simulink model "FOC_V"  (R2016b)
settings: Solver=VariableStepAuto  StartTime=0.0  StopTime=5  FixedStep=1e-6  RelTol=1e-3  EnableMultiTasking=on
model workspace (MAT data in the model file):
  Cf = 1e-05
  J = 0.02
  Lf = 0.005
  Lm = 0.27325
  Lr = 0.289368
  Ls = 0.289368
  P = 4
  Rf = 5
  Rr = 3.3278
  Rs = 4.6
  Sig = Simulink.Signal
  Sig.DataType = 'auto'
  Sig.Dimensions = -1
  Sig.DimensionsMode = 'auto'
  Sig.Complexity = 'auto'
  Sig.SampleTime = -1
  Sig.SamplingMode = 'auto'
  Ts = 0.0001
  idth = 1.6
  nth = 370
  theta0 = 0
libraries: powerlib x15, simulink x8
settings Model: Creator=yoush  LastModifiedBy=yoush
settings DataIOCC: LimitDataPoints=on
settings OptimizationCC: LifeSpan=inf
settings DebuggingCC: AllowSymbolicDim=off  SFUnexpectedBacktrackingDiag=warning  SFNoUnconditionalDefaultTransitionDiag=warning  SFExecutionAtInitializationDiag=none
settings ModelReferenceCC: PropagateSignalLabelsOutOfModel=off
settings GRTTargetCC: TargetLangStandard=C89/C90 (ANSI)
settings ConfigComp: CovMetricSettings=dw  CovHtmlReporting=on  CovSaveCumulativeToWorkspaceVar=on  CovSaveSingleToWorkspaceVar=on  CovExternalEMLEnable=off
settings ConfigurationSet: Description=SimMechanics 2G

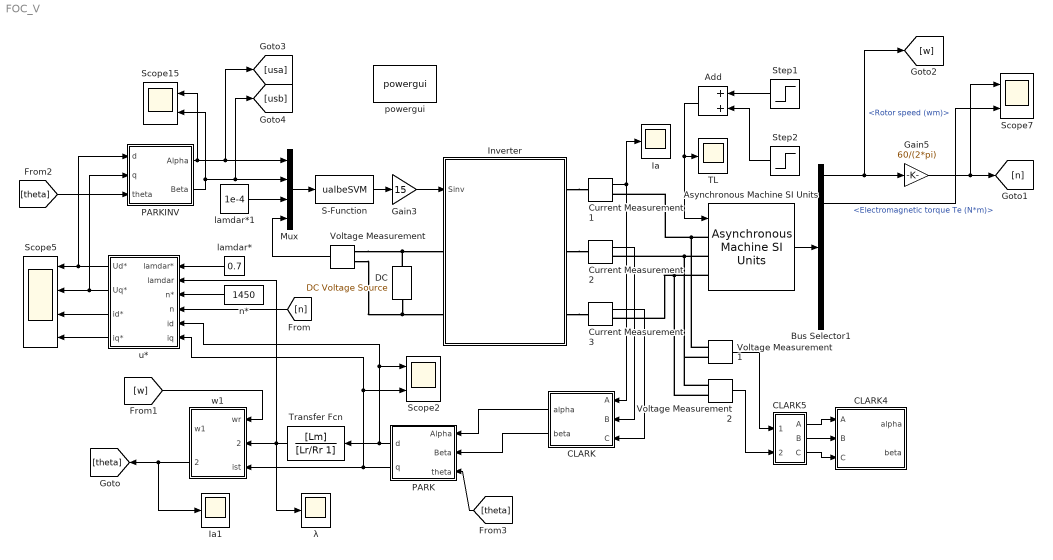
== system FOC_V ==
  Add : Sum
  Asynchronous Machine SI Units : powerlib/Machines/Asynchronous Machine SI Units  RotorType=Squirrel-cage  PresetModel=No  MechanicalLoad=Torque Tm  ShowDetailedParameters=on  ReferenceFrame=Rotor  Units=SI  MeasurementBus=off  NominalParameters=[22000 380 50]  Stator=[4.6 0.016118]  Rotor=[3.3278 0.016118]  Cage1=[0.4155 0.002066]  Cage2=[0.4168 0.0003495]  Lm=0.27325  Mechanical=[0.02 0 2]  PolePairs=2  InitialConditions=[ 1 0 0 0 0 0 0 0]  SimulateSaturation=off  Saturation=[14.03593122, 27.81365428, 53.79336849, 72.68890987, 97.98006896, 148.6815601, 215.7428561, 302.9841135, 428.7778367 ; 230, 322, 414, 460, 506, 552, 598, 644, 690]  LoadFlowParameters=1492000  TsPowergui=0  TsBlock=-1  IterativeModel=Trapezoidal non iterative  IterativeDiscreteModel=Trapezoidal non iterative  Pmec=1.492e+006
  Bus Selector1 : BusSelector  OutputSignals="Mechanical.Rotor speed (wm),Mechanical.Electromagnetic torque Te (N*m),Stator measurements.Stator current is_d (A),Stator measurements.Stator current  is_q (A),Rotor measurements.Rotor flux phir_q (V s),Rotor measurements.Rotor flux phir_d (V s)"
  CLARK : Subsystem
  CLARK4 : Subsystem
  CLARK5 : Subsystem
  Current Measurement1 : powerlib/Measurements/Current Measurement  PhasorSimulation=off  OutputType=Complex  PSBequivalent=0
  Current Measurement2 : powerlib/Measurements/Current Measurement  PhasorSimulation=off  OutputType=Complex  PSBequivalent=0
  Current Measurement3 : powerlib/Measurements/Current Measurement  PhasorSimulation=off  OutputType=Complex  PSBequivalent=0
  DC : powerlib/Electrical Sources/DC Voltage Source  Amplitude=500  Measurements=None
  Gain3 : Gain  Gain=15
  Gain5 : Gain  Gain=60/(2*pi)
  Ia : Scope
  Ia1 : Scope
  Inverter : Subsystem
  Mux : Mux
  PARK : Subsystem
  PARKINV : Subsystem
  S-Function : S-Function  FunctionName=ualbeSVM  SFunctionDeploymentMode=off  EnableBusSupport=off
  Scope15 : Scope  NumInputPorts=2
  Scope2 : Scope  NumInputPorts=2
  Scope5 : Scope  NumInputPorts=4
  Scope7 : Scope  NumInputPorts=2
  Step1 : Step  Time=2  After=2  SampleTime=0
  Step2 : Step  Time=5  After=0  SampleTime=0
  TL : Scope
  Transfer Fcn : TransferFcn  Numerator=[Lm]  Denominator=[Lr/Rr 1]
  Voltage Measurement : powerlib/Measurements/Voltage Measurement  PhasorSimulation=off  OutputType=Complex  PSBequivalent=0
  Voltage Measurement1 : powerlib/Measurements/Voltage Measurement  PhasorSimulation=off  OutputType=Complex  PSBequivalent=0
  Voltage Measurement2 : powerlib/Measurements/Voltage Measurement  PhasorSimulation=off  OutputType=Complex  PSBequivalent=0
  lamdar* : Constant  Value=0.7
  lamdar*1 : Constant  Value=1e-4
  n* : Constant  Value=1450
  powergui : powerlib/powergui  Priority=1  SimulationMode=Continuous  SolverType=Tustin/Backward Euler (TBE)  SampleTime=1e-6  frequency=60  SPID=off  DisableSnubberDevices=off  DisableRonSwitches=off  DisableVfSwitches=off  SwTol=0  DisplayEquations=off  Interpol=off  ExternalGateDelay=off  methode=off  Ts=10  FunctionMessages=off  echomessages=off  HookPort=off  EnableUseOfTLC=off  x0status=blocks  frequencyindice=50  Pbase=100e6  ErrMax=1e-4  Iterations=50  UnitsV=kV  UnitsW=MW  buscounter=0  RestoreLinks=warning  ResistiveCurrentMeasurement=off  Frange=[0:2:500]  Ylog=off  Xlog=on  ShowGrid=off  save=off  variable=ZData  structure=we  ZoomFFT=off  StartTime=0.4  cycles=5  DisplayStyle=2  fundamental=100  FreqAxis=off  MaxFrequency=1000  frequencyindicesteady=1  RmsSteady=1  display=off
  u* : Subsystem
  w1 : Subsystem
  λ : Scope
  wires:
  Current Measurement1/1 -> CLARK/1(A), Ia/1
  Add/1 -> Asynchronous Machine SI Units/1, TL/1
  Step1/1 -> Add/1
  Step2/1 -> Add/2
  Asynchronous Machine SI Units/1 -> Bus Selector1/1
  Bus Selector1/1 -> Gain5/1, [w]  "<Rotor speed (wm)>"
  Gain5/1 -> [n], Scope7/1
  Bus Selector1/2 -> Scope7/2  "<Electromagnetic torque Te (N*m)>"
  Current Measurement2/1 -> CLARK/2(B)
  Current Measurement3/1 -> CLARK/3(C)
  CLARK/1(alpha) -> PARK/1(Alpha)
  CLARK/2(beta) -> PARK/2(Beta)
  PARK/2(q) -> Scope2/2, u*/6(iq), w1/3(ist)
  [n] -> u*/4(n)
  Gain3/1 -> Inverter/1(Sinv)
  lamdar*/1 -> u*/1(lamdar*)
  n*/1 -> u*/3(n*)
  PARK/1(d) -> Transfer Fcn/1, Scope2/1, u*/5(id)
  PARKINV/1(Alpha) -> [usa], Mux/1, Scope15/1
  PARKINV/2(Beta) -> [usb], Mux/2, Scope15/2
  [theta] -> PARKINV/3(theta)
  [theta] -> PARK/3(theta)
  u*/1(Ud*) -> Scope5/1, PARKINV/1(d)
  u*/2(Uq*) -> PARKINV/2(q), Scope5/2
  Mux/1 -> S-Function/1
  lamdar*1/1 -> Mux/3
  Voltage Measurement/1 -> Mux/4
  S-Function/1 -> Gain3/1
  Transfer Fcn/1 -> λ/1, w1/2(lamdar), u*/2(lamdar)
  [w] -> w1/1(wr)
  u*/3(id*) -> Scope5/3
  w1/2(theta) -> [theta], Ia1/1
  u*/4(iq*) -> Scope5/4
  Voltage Measurement1/1 -> CLARK5/1(AB)
  Voltage Measurement2/1 -> CLARK5/2(BC)
  CLARK5/2(B) -> CLARK4/2(B)
  CLARK5/1(A) -> CLARK4/1(A)
  CLARK5/3(C) -> CLARK4/3(C)
  connections:
  Inverter/RConn1 -- Current Measurement1/LConn1
  Inverter/RConn2 -- Current Measurement2/LConn1
  Inverter/RConn3 -- Current Measurement3/LConn1
  Asynchronous Machine SI Units/LConn1 -- Voltage Measurement1/LConn1 -- Current Measurement1/RConn1
  Asynchronous Machine SI Units/LConn2 -- Voltage Measurement2/LConn1 -- Voltage Measurement1/LConn2 -- Current Measurement2/RConn1
  Asynchronous Machine SI Units/LConn3 -- Voltage Measurement2/LConn2 -- Current Measurement3/RConn1
  DC/RConn1 -- Voltage Measurement/LConn1 -- Inverter/LConn1
  DC/LConn1 -- Voltage Measurement/LConn2 -- Inverter/LConn2

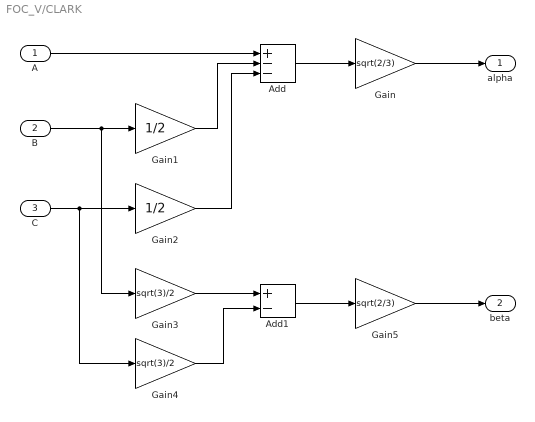
== system FOC_V/CLARK ==
  A : Inport
  B : Inport  Port=2
  C : Inport  Port=3
  Add : Sum  Inputs=+--
  Add1 : Sum  Inputs=+-
  Gain : Gain  Gain=sqrt(2/3)
  Gain1 : Gain  Gain=1/2
  Gain2 : Gain  Gain=1/2
  Gain3 : Gain  Gain=sqrt(3)/2
  Gain4 : Gain  Gain=sqrt(3)/2
  Gain5 : Gain  Gain=sqrt(2/3)
  alpha : Outport
  beta : Outport  Port=2
  wires:
  A/1 -> Add/1
  B/1 -> Gain3/1, Gain1/1
  Gain1/1 -> Add/2
  Gain2/1 -> Add/3
  C/1 -> Gain4/1, Gain2/1
  Gain3/1 -> Add1/1
  Gain4/1 -> Add1/2
  Add/1 -> Gain/1
  Add1/1 -> Gain5/1
  Gain/1 -> alpha/1
  Gain5/1 -> beta/1

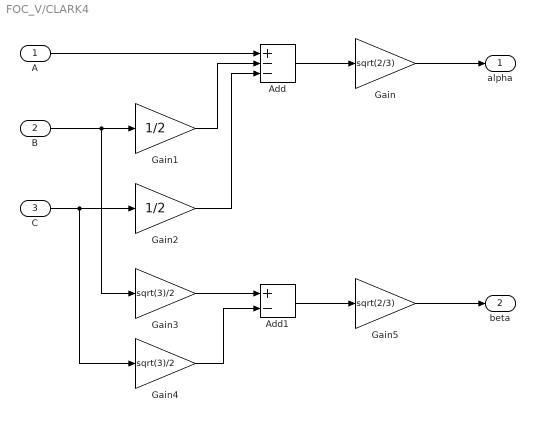
== system FOC_V/CLARK4 ==
  A : Inport
  B : Inport  Port=2
  C : Inport  Port=3
  Add : Sum  Inputs=+--
  Add1 : Sum  Inputs=+-
  Gain : Gain  Gain=sqrt(2/3)
  Gain1 : Gain  Gain=1/2
  Gain2 : Gain  Gain=1/2
  Gain3 : Gain  Gain=sqrt(3)/2
  Gain4 : Gain  Gain=sqrt(3)/2
  Gain5 : Gain  Gain=sqrt(2/3)
  alpha : Outport
  beta : Outport  Port=2
  wires:
  Gain5/1 -> beta/1
  Gain/1 -> alpha/1
  Add1/1 -> Gain5/1
  Add/1 -> Gain/1
  Gain4/1 -> Add1/2
  Gain3/1 -> Add1/1
  C/1 -> Gain2/1, Gain4/1
  Gain2/1 -> Add/3
  Gain1/1 -> Add/2
  B/1 -> Gain1/1, Gain3/1
  A/1 -> Add/1

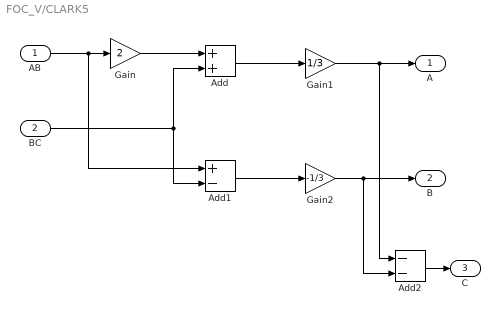
== system FOC_V/CLARK5 ==
  AB : Inport
  BC : Inport  Port=2
  Add : Sum
  Add1 : Sum  Inputs=+-
  Add2 : Sum  Inputs=--
  Gain : Gain  Gain=2
  Gain1 : Gain  Gain=1/3
  Gain2 : Gain  Gain=-1/3
  A : Outport
  B : Outport  Port=2
  C : Outport  Port=3
  wires:
  AB/1 -> Add1/1, Gain/1
  Gain/1 -> Add/1
  BC/1 -> Add/2, Add1/2
  Add/1 -> Gain1/1
  Gain1/1 -> Add2/1, A/1
  Add1/1 -> Gain2/1
  Gain2/1 -> Add2/2, B/1
  Add2/1 -> C/1

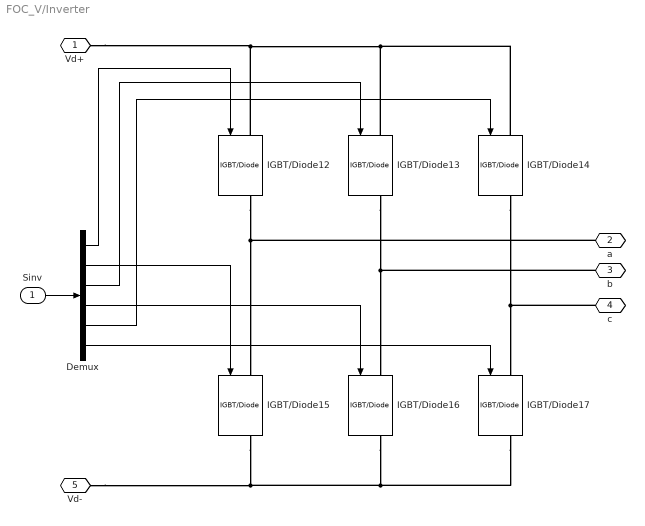
== system FOC_V/Inverter ==
  Sinv : Inport
  Demux : Demux  Outputs=6
  IGBT/Diode{12..17} (6 alike) : powerlib/Power Electronics/IGBT//Diode  Ron=1e-3  Rs=1e5  Cs=inf  Measurements=on
  Vd+ : PMIOPort  Port=1  Side=Left
  a : PMIOPort  Port=2  Side=Right
  b : PMIOPort  Port=3  Side=Right
  c : PMIOPort  Port=4  Side=Right
  Vd- : PMIOPort  Port=5  Side=Left
  wires:
  Demux/5 -> IGBT/Diode14/1
  Demux/4 -> IGBT/Diode16/1
  Demux/3 -> IGBT/Diode13/1
  Demux/6 -> IGBT/Diode17/1
  Demux/1 -> IGBT/Diode12/1
  Sinv/1 -> Demux/1
  Demux/2 -> IGBT/Diode15/1
  connections:
  IGBT/Diode12/RConn1 -- IGBT/Diode15/LConn1 -- a/RConn1
  IGBT/Diode13/RConn1 -- IGBT/Diode16/LConn1 -- b/RConn1
  IGBT/Diode14/RConn1 -- IGBT/Diode17/LConn1 -- c/RConn1
  IGBT/Diode17/RConn1 -- IGBT/Diode16/RConn1 -- Vd-/RConn1 -- IGBT/Diode15/RConn1
  IGBT/Diode12/LConn1 -- Vd+/RConn1 -- IGBT/Diode13/LConn1 -- IGBT/Diode14/LConn1

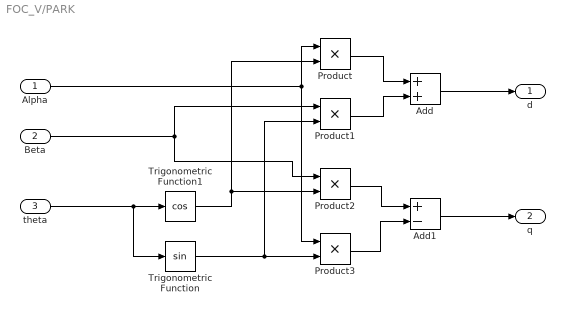
== system FOC_V/PARK ==
  Alpha : Inport
  Beta : Inport  Port=2
  theta : Inport  Port=3
  Add : Sum
  Add1 : Sum  Inputs=+-
  Product{,1..3} (4 alike) : Product
  Trigonometric Function : Trigonometry
  Trigonometric Function1 : Trigonometry  Operator=cos
  d : Outport
  q : Outport  Port=2
  wires:
  theta/1 -> Trigonometric Function1/1, Trigonometric Function/1
  Trigonometric Function1/1 -> Product/2, Product2/2
  Alpha/1 -> Product/1, Product3/1
  Trigonometric Function/1 -> Product1/2, Product3/2
  Beta/1 -> Product2/1, Product1/1
  Product/1 -> Add/1
  Product1/1 -> Add/2
  Add/1 -> d/1
  Product2/1 -> Add1/1
  Product3/1 -> Add1/2
  Add1/1 -> q/1

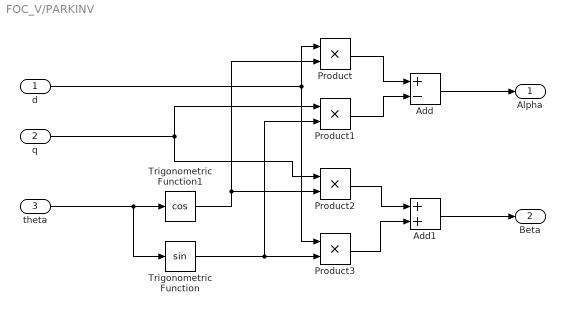
== system FOC_V/PARKINV ==
  d : Inport
  q : Inport  Port=2
  theta : Inport  Port=3
  Add : Sum  Inputs=+-
  Add1 : Sum
  Product{,1..3} (4 alike) : Product
  Trigonometric Function : Trigonometry
  Trigonometric Function1 : Trigonometry  Operator=cos
  Alpha : Outport
  Beta : Outport  Port=2
  wires:
  theta/1 -> Trigonometric Function1/1, Trigonometric Function/1
  Trigonometric Function1/1 -> Product/2, Product2/2
  d/1 -> Product/1, Product3/1
  Trigonometric Function/1 -> Product1/2, Product3/2
  q/1 -> Product2/1, Product1/1
  Product/1 -> Add/1
  Product1/1 -> Add/2
  Add/1 -> Alpha/1
  Product2/1 -> Add1/1
  Product3/1 -> Add1/2
  Add1/1 -> Beta/1

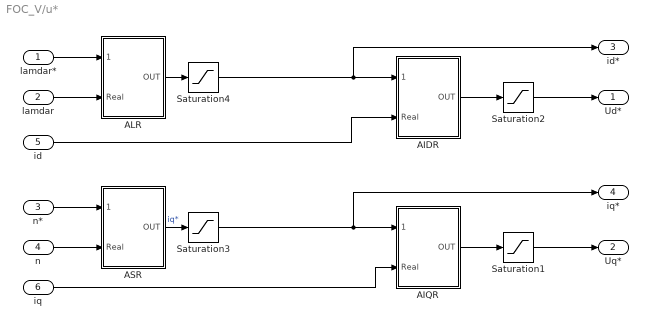
== system FOC_V/u* ==
  lamdar* : Inport
  lamdar : Inport  Port=2
  n* : Inport  Port=3
  n : Inport  Port=4
  id : Inport  Port=5
  iq : Inport  Port=6
  AIDR : Subsystem
  AIQR : Subsystem
  ALR : Subsystem
  ASR : Subsystem
  Saturation1 : Saturate  UpperLimit=380  LowerLimit=-380
  Saturation2 : Saturate  UpperLimit=380  LowerLimit=-380
  Saturation3 : Saturate  UpperLimit=5  LowerLimit=-5
  Saturation4 : Saturate  UpperLimit=5  LowerLimit=-5
  Ud* : Outport
  Uq* : Outport  Port=2
  id* : Outport  Port=3
  iq* : Outport  Port=4
  wires:
  lamdar*/1 -> ALR/1(Command)
  lamdar/1 -> ALR/2(Real)
  n*/1 -> ASR/1(Command)
  n/1 -> ASR/2(Real)
  Saturation1/1 -> Uq*/1
  Saturation2/1 -> Ud*/1
  ASR/1(OUT) -> Saturation3/1  "iq*"
  AIQR/1(OUT) -> Saturation1/1
  iq/1 -> AIQR/2(Real)
  ALR/1(OUT) -> Saturation4/1
  id/1 -> AIDR/2(Real)
  AIDR/1(OUT) -> Saturation2/1
  Saturation3/1 -> iq*/1, AIQR/1(Command)
  Saturation4/1 -> id*/1, AIDR/1(Command)

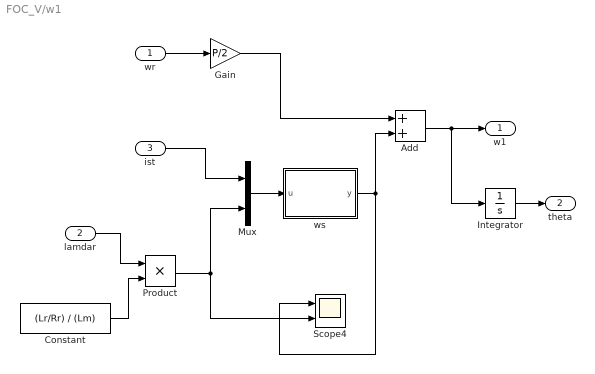
== system FOC_V/w1 ==
  wr : Inport
  lamdar : Inport  Port=2
  ist : Inport  Port=3
  Add : Sum
  Constant : Constant  Value=(Lr/Rr) / (Lm)
  Gain : Gain  Gain=P/2
  Integrator : Integrator
  Mux : Mux  Inputs=2
  Product : Product
  Scope4 : Scope  NumInputPorts=2
  ws : MATLAB Function  TreatAsAtomicUnit=on
  w1 : Outport
  theta : Outport  Port=2
  wires:
  ist/1 -> Mux/1
  Mux/1 -> ws/1(u)
  ws/1(y) -> Scope4/1, Add/2
  wr/1 -> Gain/1
  Add/1 -> Integrator/1, w1/1
  Gain/1 -> Add/1
  lamdar/1 -> Product/1
  Constant/1 -> Product/2
  Product/1 -> Mux/2, Scope4/2
  Integrator/1 -> theta/1

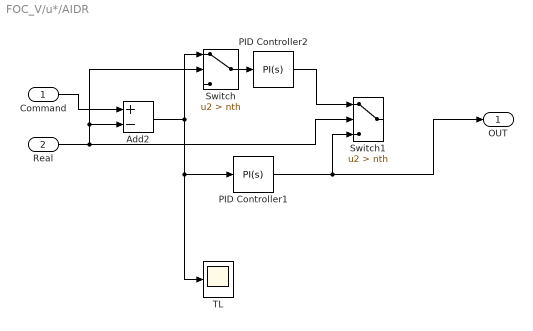
== system FOC_V/u*/AIDR ==
  Command : Inport
  Real : Inport  Port=2
  Add2 : Sum  Inputs=+-
  PID Controller1 : simulink/Continuous/PID Controller  Controller=PI  TimeDomain=Continuous-time  SampleTime=-1  IntegratorMethod=Forward Euler  FilterMethod=Forward Euler  Form=Parallel  UseFilter=on  ControllerParametersSource=internal  P=100  I=1500  D=0  N=100  InitialConditionSource=internal  InitialConditionForIntegrator=0  InitialConditionForFilter=0  ExternalReset=none  LimitOutput=off  UpperSaturationLimit=inf  LowerSaturationLimit=-inf  LinearizeAsGain=on  AntiWindupMode=none  Kb=1  TrackingMode=off  Kt=1  PParamMin=[]  PParamMax=[]  IParamMin=[]  IParamMax=[]  DParamMin=[]  DParamMax=[]  NParamMin=[]  NParamMax=[]  KbParamMin=[]  KbParamMax=[]  KtParamMin=[]  KtParamMax=[]  POutMin=[]  POutMax=[]  IOutMin=[]  IOutMax=[]  DOutMin=[]  DOutMax=[]  NOutMin=[]  NOutMax=[]  KbOutMin=[]  KbOutMax=[]  KtOutMin=[]  KtOutMax=[]  IntegratorOutMin=[]  IntegratorOutMax=[]  FilterOutMin=[]  FilterOutMax=[]  SumOutMin=[]  SumOutMax=[]  SumI1OutMin=[]  SumI1OutMax=[]  SumI2OutMin=[]  SumI2OutMax=[]  SumI3OutMin=[]  SumI3OutMax=[]  SumDOutMin=[]  SumDOutMax=[]  SaturationOutMin=[]  SaturationOutMax=[]  IntegratorContinuousStateAttributes=''  IntegratorStateMustResolveToSignalObject=off  IntegratorRTWStateStorageClass=Auto  FilterContinuousStateAttributes=''  FilterStateMustResolveToSignalObject=off  FilterRTWStateStorageClass=Auto  DifferentiatorICPrevScaledInput=0  DifferentiatorOutMin=[]  DifferentiatorOutMax=[]
  PID Controller2 : simulink/Continuous/PID Controller  Controller=PI  TimeDomain=Continuous-time  SampleTime=-1  IntegratorMethod=Forward Euler  FilterMethod=Forward Euler  Form=Parallel  UseFilter=on  ControllerParametersSource=internal  P=5  I=20  D=0  N=100  InitialConditionSource=internal  InitialConditionForIntegrator=0  InitialConditionForFilter=0  ExternalReset=none  LimitOutput=off  UpperSaturationLimit=inf  LowerSaturationLimit=-inf  LinearizeAsGain=on  AntiWindupMode=none  Kb=1  TrackingMode=off  Kt=1  PParamMin=[]  PParamMax=[]  IParamMin=[]  IParamMax=[]  DParamMin=[]  DParamMax=[]  NParamMin=[]  NParamMax=[]  KbParamMin=[]  KbParamMax=[]  KtParamMin=[]  KtParamMax=[]  POutMin=[]  POutMax=[]  IOutMin=[]  IOutMax=[]  DOutMin=[]  DOutMax=[]  NOutMin=[]  NOutMax=[]  KbOutMin=[]  KbOutMax=[]  KtOutMin=[]  KtOutMax=[]  IntegratorOutMin=[]  IntegratorOutMax=[]  FilterOutMin=[]  FilterOutMax=[]  SumOutMin=[]  SumOutMax=[]  SumI1OutMin=[]  SumI1OutMax=[]  SumI2OutMin=[]  SumI2OutMax=[]  SumI3OutMin=[]  SumI3OutMax=[]  SumDOutMin=[]  SumDOutMax=[]  SaturationOutMin=[]  SaturationOutMax=[]  IntegratorContinuousStateAttributes=''  IntegratorStateMustResolveToSignalObject=off  IntegratorRTWStateStorageClass=Auto  FilterContinuousStateAttributes=''  FilterStateMustResolveToSignalObject=off  FilterRTWStateStorageClass=Auto  DifferentiatorICPrevScaledInput=0  DifferentiatorOutMin=[]  DifferentiatorOutMax=[]
  Switch : Switch  Criteria=u2 > Threshold  Threshold=nth
  Switch1 : Switch  Criteria=u2 > Threshold  Threshold=nth
  TL : Scope
  OUT : Outport
  wires:
  PID Controller1/1 -> Switch1/3, OUT/1
  PID Controller2/1 -> Switch1/1
  Switch/1 -> PID Controller2/1
  Add2/1 -> PID Controller1/1, TL/1, Switch/1
  Command/1 -> Add2/1
  Real/1 -> Switch1/2, Switch/2, Add2/2

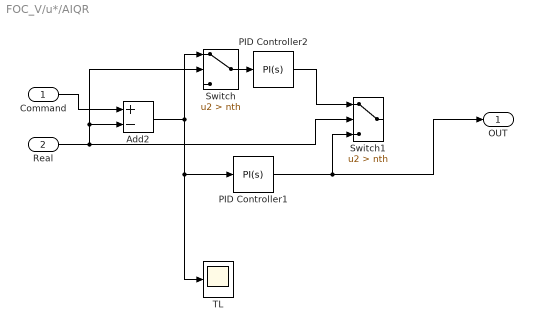
== system FOC_V/u*/AIQR ==
  Command : Inport
  Real : Inport  Port=2
  Add2 : Sum  Inputs=+-
  PID Controller1 : simulink/Continuous/PID Controller  Controller=PI  TimeDomain=Continuous-time  SampleTime=-1  IntegratorMethod=Forward Euler  FilterMethod=Forward Euler  Form=Parallel  UseFilter=on  ControllerParametersSource=internal  P=50  I=1000  D=0  N=100  InitialConditionSource=internal  InitialConditionForIntegrator=0  InitialConditionForFilter=0  ExternalReset=none  LimitOutput=off  UpperSaturationLimit=inf  LowerSaturationLimit=-inf  LinearizeAsGain=on  AntiWindupMode=none  Kb=1  TrackingMode=off  Kt=1  PParamMin=[]  PParamMax=[]  IParamMin=[]  IParamMax=[]  DParamMin=[]  DParamMax=[]  NParamMin=[]  NParamMax=[]  KbParamMin=[]  KbParamMax=[]  KtParamMin=[]  KtParamMax=[]  POutMin=[]  POutMax=[]  IOutMin=[]  IOutMax=[]  DOutMin=[]  DOutMax=[]  NOutMin=[]  NOutMax=[]  KbOutMin=[]  KbOutMax=[]  KtOutMin=[]  KtOutMax=[]  IntegratorOutMin=[]  IntegratorOutMax=[]  FilterOutMin=[]  FilterOutMax=[]  SumOutMin=[]  SumOutMax=[]  SumI1OutMin=[]  SumI1OutMax=[]  SumI2OutMin=[]  SumI2OutMax=[]  SumI3OutMin=[]  SumI3OutMax=[]  SumDOutMin=[]  SumDOutMax=[]  SaturationOutMin=[]  SaturationOutMax=[]  IntegratorContinuousStateAttributes=''  IntegratorStateMustResolveToSignalObject=off  IntegratorRTWStateStorageClass=Auto  FilterContinuousStateAttributes=''  FilterStateMustResolveToSignalObject=off  FilterRTWStateStorageClass=Auto  DifferentiatorICPrevScaledInput=0  DifferentiatorOutMin=[]  DifferentiatorOutMax=[]
  PID Controller2 : simulink/Continuous/PID Controller  Controller=PI  TimeDomain=Continuous-time  SampleTime=-1  IntegratorMethod=Forward Euler  FilterMethod=Forward Euler  Form=Parallel  UseFilter=on  ControllerParametersSource=internal  P=5  I=20  D=0  N=100  InitialConditionSource=internal  InitialConditionForIntegrator=0  InitialConditionForFilter=0  ExternalReset=none  LimitOutput=off  UpperSaturationLimit=inf  LowerSaturationLimit=-inf  LinearizeAsGain=on  AntiWindupMode=none  Kb=1  TrackingMode=off  Kt=1  PParamMin=[]  PParamMax=[]  IParamMin=[]  IParamMax=[]  DParamMin=[]  DParamMax=[]  NParamMin=[]  NParamMax=[]  KbParamMin=[]  KbParamMax=[]  KtParamMin=[]  KtParamMax=[]  POutMin=[]  POutMax=[]  IOutMin=[]  IOutMax=[]  DOutMin=[]  DOutMax=[]  NOutMin=[]  NOutMax=[]  KbOutMin=[]  KbOutMax=[]  KtOutMin=[]  KtOutMax=[]  IntegratorOutMin=[]  IntegratorOutMax=[]  FilterOutMin=[]  FilterOutMax=[]  SumOutMin=[]  SumOutMax=[]  SumI1OutMin=[]  SumI1OutMax=[]  SumI2OutMin=[]  SumI2OutMax=[]  SumI3OutMin=[]  SumI3OutMax=[]  SumDOutMin=[]  SumDOutMax=[]  SaturationOutMin=[]  SaturationOutMax=[]  IntegratorContinuousStateAttributes=''  IntegratorStateMustResolveToSignalObject=off  IntegratorRTWStateStorageClass=Auto  FilterContinuousStateAttributes=''  FilterStateMustResolveToSignalObject=off  FilterRTWStateStorageClass=Auto  DifferentiatorICPrevScaledInput=0  DifferentiatorOutMin=[]  DifferentiatorOutMax=[]
  Switch : Switch  Criteria=u2 > Threshold  Threshold=nth
  Switch1 : Switch  Criteria=u2 > Threshold  Threshold=nth
  TL : Scope
  OUT : Outport
  wires:
  Real/1 -> Add2/2, Switch/2, Switch1/2
  Command/1 -> Add2/1
  Add2/1 -> Switch/1, TL/1, PID Controller1/1
  Switch/1 -> PID Controller2/1
  PID Controller2/1 -> Switch1/1
  PID Controller1/1 -> OUT/1, Switch1/3

== system FOC_V/u*/ALR ==
  Command : Inport
  Real : Inport  Port=2
  Add2 : Sum  Inputs=+-
  PID Controller1 : simulink/Continuous/PID Controller  Controller=PI  TimeDomain=Continuous-time  SampleTime=-1  IntegratorMethod=Forward Euler  FilterMethod=Forward Euler  Form=Parallel  UseFilter=on  ControllerParametersSource=internal  P=50  I=120  D=0  N=100  InitialConditionSource=internal  InitialConditionForIntegrator=0  InitialConditionForFilter=0  ExternalReset=none  LimitOutput=off  UpperSaturationLimit=inf  LowerSaturationLimit=-inf  LinearizeAsGain=on  AntiWindupMode=none  Kb=1  TrackingMode=off  Kt=1  PParamMin=[]  PParamMax=[]  IParamMin=[]  IParamMax=[]  DParamMin=[]  DParamMax=[]  NParamMin=[]  NParamMax=[]  KbParamMin=[]  KbParamMax=[]  KtParamMin=[]  KtParamMax=[]  POutMin=[]  POutMax=[]  IOutMin=[]  IOutMax=[]  DOutMin=[]  DOutMax=[]  NOutMin=[]  NOutMax=[]  KbOutMin=[]  KbOutMax=[]  KtOutMin=[]  KtOutMax=[]  IntegratorOutMin=[]  IntegratorOutMax=[]  FilterOutMin=[]  FilterOutMax=[]  SumOutMin=[]  SumOutMax=[]  SumI1OutMin=[]  SumI1OutMax=[]  SumI2OutMin=[]  SumI2OutMax=[]  SumI3OutMin=[]  SumI3OutMax=[]  SumDOutMin=[]  SumDOutMax=[]  SaturationOutMin=[]  SaturationOutMax=[]  IntegratorContinuousStateAttributes=''  IntegratorStateMustResolveToSignalObject=off  IntegratorRTWStateStorageClass=Auto  FilterContinuousStateAttributes=''  FilterStateMustResolveToSignalObject=off  FilterRTWStateStorageClass=Auto  DifferentiatorICPrevScaledInput=0  DifferentiatorOutMin=[]  DifferentiatorOutMax=[]
  PID Controller2 : simulink/Continuous/PID Controller  Controller=PI  TimeDomain=Continuous-time  SampleTime=-1  IntegratorMethod=Forward Euler  FilterMethod=Forward Euler  Form=Parallel  UseFilter=on  ControllerParametersSource=internal  P=20  I=200  D=0  N=100  InitialConditionSource=internal  InitialConditionForIntegrator=0  InitialConditionForFilter=0  ExternalReset=none  LimitOutput=off  UpperSaturationLimit=inf  LowerSaturationLimit=-inf  LinearizeAsGain=on  AntiWindupMode=none  Kb=1  TrackingMode=off  Kt=1  PParamMin=[]  PParamMax=[]  IParamMin=[]  IParamMax=[]  DParamMin=[]  DParamMax=[]  NParamMin=[]  NParamMax=[]  KbParamMin=[]  KbParamMax=[]  KtParamMin=[]  KtParamMax=[]  POutMin=[]  POutMax=[]  IOutMin=[]  IOutMax=[]  DOutMin=[]  DOutMax=[]  NOutMin=[]  NOutMax=[]  KbOutMin=[]  KbOutMax=[]  KtOutMin=[]  KtOutMax=[]  IntegratorOutMin=[]  IntegratorOutMax=[]  FilterOutMin=[]  FilterOutMax=[]  SumOutMin=[]  SumOutMax=[]  SumI1OutMin=[]  SumI1OutMax=[]  SumI2OutMin=[]  SumI2OutMax=[]  SumI3OutMin=[]  SumI3OutMax=[]  SumDOutMin=[]  SumDOutMax=[]  SaturationOutMin=[]  SaturationOutMax=[]  IntegratorContinuousStateAttributes=''  IntegratorStateMustResolveToSignalObject=off  IntegratorRTWStateStorageClass=Auto  FilterContinuousStateAttributes=''  FilterStateMustResolveToSignalObject=off  FilterRTWStateStorageClass=Auto  DifferentiatorICPrevScaledInput=0  DifferentiatorOutMin=[]  DifferentiatorOutMax=[]
  Switch : Switch  Criteria=u2 > Threshold  Threshold=idth
  Switch1 : Switch  Criteria=u2 > Threshold  Threshold=idth
  error : Scope
  OUT : Outport
  wires:
  PID Controller2/1 -> Switch1/1
  Switch/1 -> PID Controller2/1
  Add2/1 -> error/1, PID Controller1/1, Switch/1
  Command/1 -> Add2/1
  Real/1 -> Switch1/2, Switch/2, Add2/2
  PID Controller1/1 -> OUT/1

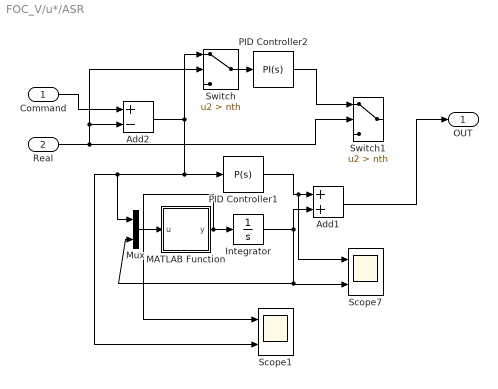
== system FOC_V/u*/ASR ==
  Command : Inport
  Real : Inport  Port=2
  Add1 : Sum
  Add2 : Sum  Inputs=+-
  Integrator : Integrator
  MATLAB Function : MATLAB Function  TreatAsAtomicUnit=on
  Mux : Mux  Inputs=2
  PID Controller1 : simulink/Continuous/PID Controller  Controller=P  TimeDomain=Continuous-time  SampleTime=-1  IntegratorMethod=Forward Euler  FilterMethod=Forward Euler  Form=Parallel  UseFilter=on  ControllerParametersSource=internal  P=1  I=20  D=0  N=100  InitialConditionSource=internal  InitialConditionForIntegrator=0  InitialConditionForFilter=0  ExternalReset=none  LimitOutput=off  UpperSaturationLimit=inf  LowerSaturationLimit=-inf  LinearizeAsGain=on  AntiWindupMode=none  Kb=1  TrackingMode=off  Kt=1  PParamMin=[]  PParamMax=[]  IParamMin=[]  IParamMax=[]  DParamMin=[]  DParamMax=[]  NParamMin=[]  NParamMax=[]  KbParamMin=[]  KbParamMax=[]  KtParamMin=[]  KtParamMax=[]  POutMin=[]  POutMax=[]  IOutMin=[]  IOutMax=[]  DOutMin=[]  DOutMax=[]  NOutMin=[]  NOutMax=[]  KbOutMin=[]  KbOutMax=[]  KtOutMin=[]  KtOutMax=[]  IntegratorOutMin=[]  IntegratorOutMax=[]  FilterOutMin=[]  FilterOutMax=[]  SumOutMin=[]  SumOutMax=[]  SumI1OutMin=[]  SumI1OutMax=[]  SumI2OutMin=[]  SumI2OutMax=[]  SumI3OutMin=[]  SumI3OutMax=[]  SumDOutMin=[]  SumDOutMax=[]  SaturationOutMin=[]  SaturationOutMax=[]  IntegratorContinuousStateAttributes=''  IntegratorStateMustResolveToSignalObject=off  IntegratorRTWStateStorageClass=Auto  FilterContinuousStateAttributes=''  FilterStateMustResolveToSignalObject=off  FilterRTWStateStorageClass=Auto  DifferentiatorICPrevScaledInput=0  DifferentiatorOutMin=[]  DifferentiatorOutMax=[]
  PID Controller2 : simulink/Continuous/PID Controller  Controller=PI  TimeDomain=Continuous-time  SampleTime=-1  IntegratorMethod=Forward Euler  FilterMethod=Forward Euler  Form=Parallel  UseFilter=on  ControllerParametersSource=internal  P=10  I=100  D=0  N=100  InitialConditionSource=internal  InitialConditionForIntegrator=0  InitialConditionForFilter=0  ExternalReset=none  LimitOutput=off  UpperSaturationLimit=inf  LowerSaturationLimit=-inf  LinearizeAsGain=on  AntiWindupMode=none  Kb=1  TrackingMode=off  Kt=1  PParamMin=[]  PParamMax=[]  IParamMin=[]  IParamMax=[]  DParamMin=[]  DParamMax=[]  NParamMin=[]  NParamMax=[]  KbParamMin=[]  KbParamMax=[]  KtParamMin=[]  KtParamMax=[]  POutMin=[]  POutMax=[]  IOutMin=[]  IOutMax=[]  DOutMin=[]  DOutMax=[]  NOutMin=[]  NOutMax=[]  KbOutMin=[]  KbOutMax=[]  KtOutMin=[]  KtOutMax=[]  IntegratorOutMin=[]  IntegratorOutMax=[]  FilterOutMin=[]  FilterOutMax=[]  SumOutMin=[]  SumOutMax=[]  SumI1OutMin=[]  SumI1OutMax=[]  SumI2OutMin=[]  SumI2OutMax=[]  SumI3OutMin=[]  SumI3OutMax=[]  SumDOutMin=[]  SumDOutMax=[]  SaturationOutMin=[]  SaturationOutMax=[]  IntegratorContinuousStateAttributes=''  IntegratorStateMustResolveToSignalObject=off  IntegratorRTWStateStorageClass=Auto  FilterContinuousStateAttributes=''  FilterStateMustResolveToSignalObject=off  FilterRTWStateStorageClass=Auto  DifferentiatorICPrevScaledInput=0  DifferentiatorOutMin=[]  DifferentiatorOutMax=[]
  Scope1 : Scope  NumInputPorts=2
  Scope7 : Scope  NumInputPorts=2
  Switch : Switch  Criteria=u2 > Threshold  Threshold=nth
  Switch1 : Switch  Criteria=u2 > Threshold  Threshold=nth
  OUT : Outport
  wires:
  Real/1 -> Add2/2, Switch/2, Switch1/2
  Command/1 -> Add2/1
  Add2/1 -> Switch/1, Mux/1, Scope1/2, PID Controller1/1
  Switch/1 -> PID Controller2/1
  PID Controller2/1 -> Switch1/1
  Integrator/1 -> Mux/2, Scope7/2, Add1/2
  PID Controller1/1 -> Scope7/1, Add1/1
  Add1/1 -> OUT/1
  MATLAB Function/1(y) -> Scope1/1, Integrator/1
  Mux/1 -> MATLAB Function/1(u)

== matlab function FOC_V/u*/ASR/MATLAB Function ==
  data: u input; y output
function y = fcn(u)
if u(2) > 20 && u(1) > 0
    y = 0;
else
    y = 5 * u(1);
end

== matlab function FOC_V/w1/ws ==
  data: u input; y output
function y = fcn(u)
if (u(2) > 0.01)
    y = u(1) / u(2);
else
    y = 0;
end
